simulink model "Kalman_gefiltert"  (R2019b)
settings: Solver=FixedStepAuto  StartTime=0.0  StopTime=sim  FixedStep=1  RelTol=1e-3
undefined symbols (not defined in the file or in its folder): DATA013punkte, Discrete, Time
libraries: ctrlSharedLib x1

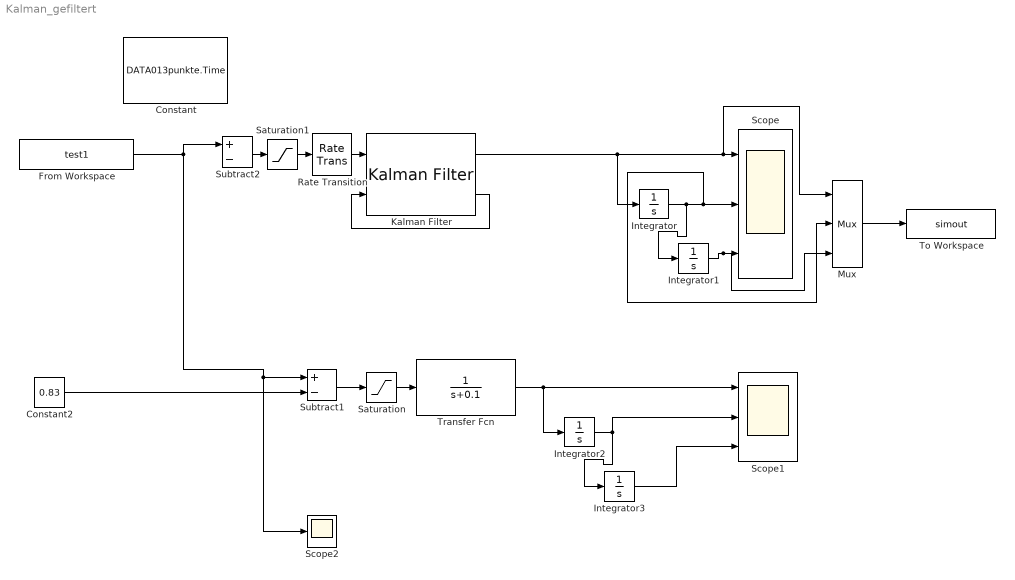
== system Kalman_gefiltert ==
  Constant : Constant  Value=DATA013punkte.Time
  Constant2 : Constant  Value=0.83
  From Workspace : FromWorkspace  VariableName=test1  SampleTime=0
  Integrator{,1..3} (4 alike) : Integrator
  Kalman Filter : ctrlSharedLib/Kalman Filter  TimeDomain=Discrete-Time  UseCurrentEstimator=on  ModelSource=LTI State-Space Variable  ModelSourceVariable=ss(0.95,1,1,0,1)  A=0.95  B=1  C=1  D=0  NumberOfStates=1  NumberOfInputs=1  NumberOfOutputs=1  InitialEstimateSource=Dialog  X0=0  P0=10  UseK=off  UseGH=off  NumberOfProcessNoiseInputs=1  G=1  TimeInvariantG=on  H=0  TimeInvariantH=on  Q=0.05  TimeInvariantQ=on  R=1  TimeInvariantR=on  N=0  TimeInvariantN=on  AddInputPort=on  AddEnablePort=off  OutputEstimatedY=on  OutputP=off  Ts=-1
  Mux : Mux  Inputs=3
  Rate Transition : RateTransition
  Saturation : Saturate  UpperLimit=inf  LowerLimit=-inf
  Saturation1 : Saturate  UpperLimit=inf  LowerLimit=0
  Scope : Scope  NumInputPorts=3
  Scope1 : Scope  NumInputPorts=3
  Scope2 : Scope
  Subtract1 : Sum  Inputs=+-
  Subtract2 : Sum  Inputs=+-
  To Workspace : ToWorkspace  VariableName=simout  SaveFormat=Timeseries  SampleTime=-1
  Transfer Fcn : TransferFcn  Denominator=[1 0.1]
  wires:
  Kalman Filter/2 -> Kalman Filter/2
  Rate Transition/1 -> Kalman Filter/1
  Kalman Filter/1 -> Integrator/1, Mux/1, Scope/1
  Integrator/1 -> Integrator1/1, Scope/2, Mux/2
  Integrator1/1 -> Mux/3, Scope/3
  Integrator3/1 -> Scope1/3
  Transfer Fcn/1 -> Integrator2/1, Scope1/1
  Integrator2/1 -> Integrator3/1, Scope1/2
  Subtract1/1 -> Saturation/1
  Saturation/1 -> Transfer Fcn/1
  Subtract2/1 -> Saturation1/1
  Constant2/1 -> Subtract1/2
  From Workspace/1 -> Subtract2/1, Scope2/1, Subtract1/1
  Saturation1/1 -> Rate Transition/1
  Mux/1 -> To Workspace/1
